simulink model "Ex2Week1Simupdate"  (R2023b)
settings: Solver=VariableStepAuto  StartTime=0.0  StopTime=10  RelTol=1e-9
settings Model: Creator=andyjwaideh  LastModifiedBy=aliawolken

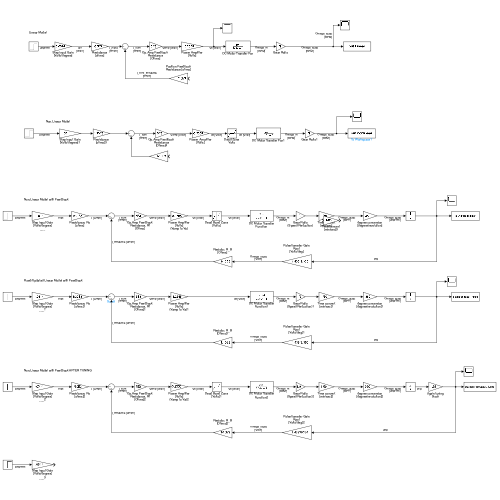
[thumbnail: Simulink's stored preview of the top-level diagram]
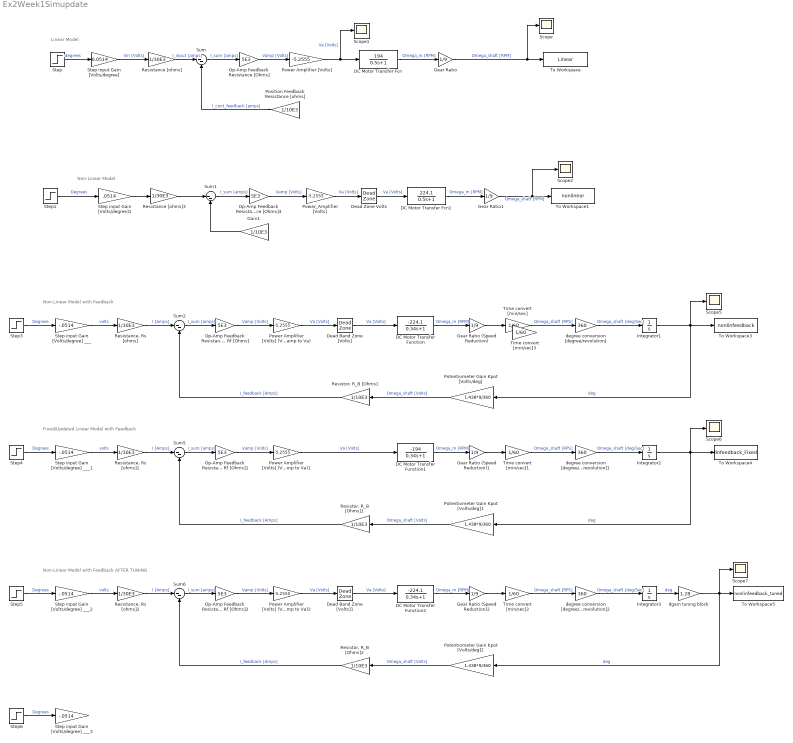
== system Ex2Week1Simupdate ==
  note: Non-Linear Model
  note: Linear Model
  note: Non-Linear Model with Feedback
  note: Fixed/Updated Linear Model with Feedback
  note: Non-Linear Model with Feedback AFTER TUNING
  DC Motor Transfer Function : TransferFcn  Numerator=[-224.1]  Denominator=[0.34 1]
  DC Motor Transfer Function1 : TransferFcn  Numerator=[-194]  Denominator=[0.34 1]
  DC Motor Transfer Function2 : TransferFcn  Numerator=[-224.1]  Denominator=[0.34 1]
  DC Motor Transfer Fcn : TransferFcn  Numerator=[194]  Denominator=[0.5 1]
  DC Motor Transfer Fcn1 : TransferFcn  Numerator=[224.1]  Denominator=[0.5 1]
  Dead Band Zone [Volts] : DeadZone  LowerValue=-1.23  UpperValue=1.23
  Dead Band Zone [Volts]1 : DeadZone  LowerValue=-1.23  UpperValue=1.23
  Dead Zone Volts : DeadZone  LowerValue=-1  UpperValue=1
  Gain1 : Gain  Gain=1/10E3
  Gear Ratio : Gain  Gain=1/9
  Gear Ratio (Speed Reduction) : Gain  Gain=1/9
  Gear Ratio (Speed Reduction)1 : Gain  Gain=1/9
  Gear Ratio (Speed Reduction)2 : Gain  Gain=1/9
  Gear Ratio1 : Gain  Gain=1/9
  Integrator1 : Integrator
  Integrator2 : Integrator
  Integrator3 : Integrator
  Op-Amp Feedback Resistance [Ohms] : Gain  Gain=5E3
  Op-Amp Feedback Resistance [Ohms]4 : Gain  Gain=5E3
  "Op-Amp Feedback Resistance, Rf [Ohms]" : Gain  Gain=5E3
  "Op-Amp Feedback Resistance, Rf [Ohms]1" : Gain  Gain=5E3
  "Op-Amp Feedback Resistance, Rf [Ohms]2" : Gain  Gain=5E3
  Position Feedback Resistance [ohms] : Gain  Gain=1/10E3
  Potentiometer Gain Kpot [Volts/deg] : Gain  Gain=1.438*9/360
  Potentiometer Gain Kpot [Volts/deg]1 : Gain  Gain=1.438*9/360
  Potentiometer Gain Kpot [Volts/deg]2 : Gain  Gain=1.438*9/360
  Power Amplifier [Volts] : Gain  Gain=-5.2555
  Power Amplifier [Volts] (Vamp to Va) : Gain  Gain=-5.2555
  Power Amplifier [Volts] (Vamp to Va)1 : Gain  Gain=-5.2555
  Power Amplifier [Volts] (Vamp to Va)2 : Gain  Gain=-5.2555
  Power_Amplifier [Volts] : Gain  Gain=-5.2555
  Resistance [ohms] : Gain  Gain=1/30E3
  Resistance [ohms]3 : Gain  Gain=1/30E3
  "Resistance, Rs [ohms]" : Gain  Gain=1/30E3
  "Resistance, Rs [ohms]1" : Gain  Gain=1/30E3
  "Resistance, Rs [ohms]2" : Gain  Gain=1/30E3
  "Resistor, R_B [Ohms]" : Gain  Gain=1/10E3
  "Resistor, R_B [Ohms]1" : Gain  Gain=1/10E3
  "Resistor, R_B [Ohms]2" : Gain  Gain=1/10E3
  Scope{,1..2,5..7} (6 alike) : Scope
  Step{,1,3..6} (6 alike) : Step  After=180  SampleTime=0
  Step input Gain [Volts/degree] : Gain  Gain=0.0514
  Step input Gain [Volts/degree] ___{,1..3} (4 alike) : Gain  Gain=-.0514
  Step input Gain [Volts/degree]1 : Gain  Gain=.0514
  Sum{,1..2,5..6} (5 alike) : Sum  Inputs=|--
  Time convert [min/sec]{,1..3} (4 alike) : Gain  Gain=1/60
  To Workspace : ToWorkspace  VariableName=Linear  SampleTime=-1
  To Workspace1 : ToWorkspace  VariableName=nonlinear  SampleTime=-1
  To Workspace3 : ToWorkspace  VariableName=nonlinfeedback  SampleTime=-1
  To Workspace4 : ToWorkspace  VariableName=linfeedback_Fixed  SampleTime=-1
  To Workspace5 : ToWorkspace  VariableName=nonlinfeedback_tuned  SampleTime=-1
  degree conversion [degree/revolution] : Gain  Gain=360
  degree conversion [degree/revolution]1 : Gain  Gain=360
  degree conversion [degree/revolution]2 : Gain  Gain=360
  dgain tuning block : Gain  Gain=1.28
  wires:
  Step1/1 -> Step input Gain [Volts/degree]1/1  "Degrees"
  Power Amplifier [Volts]/1 -> Scope1/1, DC Motor Transfer Fcn/1  "Va [Volts]"
  DC Motor Transfer Fcn/1 -> Gear Ratio/1  "Omega_m [RPM]"
  Gear Ratio/1 -> Scope/1, To Workspace/1  "Omega_shaft [RPM]"
  DC Motor Transfer Fcn1/1 -> Gear Ratio1/1  "Omega_m [RPM]"
  Power_Amplifier [Volts]/1 -> Dead Zone Volts/1  "Va [Volts]"
  Dead Zone Volts/1 -> DC Motor Transfer Fcn1/1  "Va [Volts]"
  Step/1 -> Step input Gain [Volts/degree]/1  "degrees"
  Resistance [ohms]/1 -> Sum/1  "I_input [amps]"
  Op-Amp Feedback Resistance [Ohms]/1 -> Power Amplifier [Volts]/1  "Vamp [Volts]"
  Sum/1 -> Op-Amp Feedback Resistance [Ohms]/1  "I_sum [amps]"
  Position Feedback Resistance [ohms]/1 -> Sum/2  "I_cont_feedback [amps]"
  Gain1/1 -> Sum1/2
  Sum1/1 -> Op-Amp Feedback Resistance [Ohms]4/1  "I_sum [amps]"
  Op-Amp Feedback Resistance [Ohms]4/1 -> Power_Amplifier [Volts]/1  "Vamp [Volts]"
  Resistance [ohms]3/1 -> Sum1/1
  Gear Ratio1/1 -> Scope2/1, To Workspace1/1  "Omega_shaft [RPM]"
  Step input Gain [Volts/degree]1/1 -> Resistance [ohms]3/1
  Step input Gain [Volts/degree]/1 -> Resistance [ohms]/1  "Vin [Volts]"
  Gear Ratio (Speed Reduction)/1 -> Time convert [min/sec]/1
  "Resistance, Rs [ohms]"/1 -> Sum2/1  "I [Amps]"
  "Op-Amp Feedback Resistance, Rf [Ohms]"/1 -> Power Amplifier [Volts] (Vamp to Va)/1  "Vamp [Volts]"
  Sum2/1 -> "Op-Amp Feedback Resistance, Rf [Ohms]"/1  "I_sum [amps]"
  "Resistor, R_B [Ohms]"/1 -> Sum2/2  "I_feedback [Amps]"
  Dead Band Zone [Volts]/1 -> DC Motor Transfer Function/1  "Va [Volts]"
  Power Amplifier [Volts] (Vamp to Va)/1 -> Dead Band Zone [Volts]/1  "Va [Volts]"
  DC Motor Transfer Function/1 -> Gear Ratio (Speed Reduction)/1  "Omega_m [RPM]"
  Step3/1 -> Step input Gain [Volts/degree] ___/1  "Degrees"
  Step input Gain [Volts/degree] ___/1 -> "Resistance, Rs [ohms]"/1  "volts"
  Potentiometer Gain Kpot [Volts/deg]/1 -> "Resistor, R_B [Ohms]"/1  "Omega_shaft [Volts]"
  Integrator1/1 -> To Workspace3/1, Potentiometer Gain Kpot [Volts/deg]/1, Scope5/1  "deg"
  Time convert [min/sec]/1 -> degree conversion [degree/revolution]/1  "Omega_shaft [RPS]"
  degree conversion [degree/revolution]/1 -> Integrator1/1  "Omega_shaft [deg/Sec]"
  "Resistance, Rs [ohms]1"/1 -> Sum5/1  "I [Amps]"
  Gear Ratio (Speed Reduction)1/1 -> Time convert [min/sec]1/1
  "Op-Amp Feedback Resistance, Rf [Ohms]1"/1 -> Power Amplifier [Volts] (Vamp to Va)1/1  "Vamp [Volts]"
  Step4/1 -> Step input Gain [Volts/degree] ___1/1  "Degrees"
  Power Amplifier [Volts] (Vamp to Va)1/1 -> DC Motor Transfer Function1/1  "Va [Volts]"
  Step input Gain [Volts/degree] ___1/1 -> "Resistance, Rs [ohms]1"/1  "volts"
  DC Motor Transfer Function1/1 -> Gear Ratio (Speed Reduction)1/1  "Omega_m [RPM]"
  Sum5/1 -> "Op-Amp Feedback Resistance, Rf [Ohms]1"/1  "I_sum [amps]"
  Potentiometer Gain Kpot [Volts/deg]1/1 -> "Resistor, R_B [Ohms]1"/1  "Omega_shaft [Volts]"
  "Resistor, R_B [Ohms]1"/1 -> Sum5/2  "I_feedback [Amps]"
  Integrator2/1 -> To Workspace4/1, Potentiometer Gain Kpot [Volts/deg]1/1, Scope6/1  "deg"
  Time convert [min/sec]1/1 -> degree conversion [degree/revolution]1/1  "Omega_shaft [RPS]"
  degree conversion [degree/revolution]1/1 -> Integrator2/1  "Omega_shaft [deg/Sec]"
  "Resistance, Rs [ohms]2"/1 -> Sum6/1  "I [Amps]"
  Gear Ratio (Speed Reduction)2/1 -> Time convert [min/sec]2/1
  "Op-Amp Feedback Resistance, Rf [Ohms]2"/1 -> Power Amplifier [Volts] (Vamp to Va)2/1  "Vamp [Volts]"
  Power Amplifier [Volts] (Vamp to Va)2/1 -> Dead Band Zone [Volts]1/1  "Va [Volts]"
  Step5/1 -> Step input Gain [Volts/degree] ___2/1  "Degrees"
  Dead Band Zone [Volts]1/1 -> DC Motor Transfer Function2/1  "Va [Volts]"
  Step input Gain [Volts/degree] ___2/1 -> "Resistance, Rs [ohms]2"/1  "volts"
  DC Motor Transfer Function2/1 -> Gear Ratio (Speed Reduction)2/1  "Omega_m [RPM]"
  Sum6/1 -> "Op-Amp Feedback Resistance, Rf [Ohms]2"/1  "I_sum [amps]"
  Potentiometer Gain Kpot [Volts/deg]2/1 -> "Resistor, R_B [Ohms]2"/1  "Omega_shaft [Volts]"
  "Resistor, R_B [Ohms]2"/1 -> Sum6/2  "I_feedback [Amps]"
  Integrator3/1 -> dgain tuning block/1  "deg"
  Time convert [min/sec]2/1 -> degree conversion [degree/revolution]2/1  "Omega_shaft [RPS]"
  degree conversion [degree/revolution]2/1 -> Integrator3/1  "Omega_shaft [deg/Sec]"
  dgain tuning block/1 -> To Workspace5/1, Potentiometer Gain Kpot [Volts/deg]2/1, Scope7/1  "deg"
  Step6/1 -> Step input Gain [Volts/degree] ___3/1  "Degrees"
